simulink model "LQG"  (R2023a)
settings: Solver=FixedStepDiscrete  StartTime=0.0  StopTime=input_settings.flight_time  FixedStep=input_settings.dt  RelTol=1e-3
undefined symbols (not defined in the file): control_surface_mapping, DiscIntNeverNeededParam, Discrete, input_settings, linear_sys, LQR_gain, Rn, saturation_deflection_rate, sys_kf, Time
libraries: ctrlSharedLib x1
settings Model: Creator=sjd320  LastModifiedBy=sduess
settings DebuggingCC: UnconnectedInputMsg=warning  UnconnectedOutputMsg=warning  UnconnectedLineMsg=warning
settings ModelReferenceCC: EnableRefExpFcnMdlSchedulingChecks=on
settings RTWCC: DLArmComputeVersion=19.05

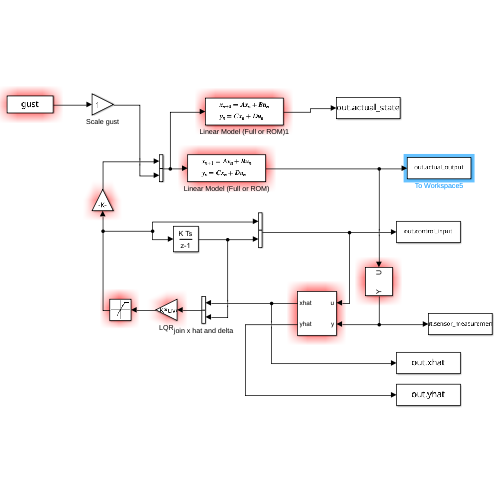
[thumbnail: Simulink's stored preview of the top-level diagram]
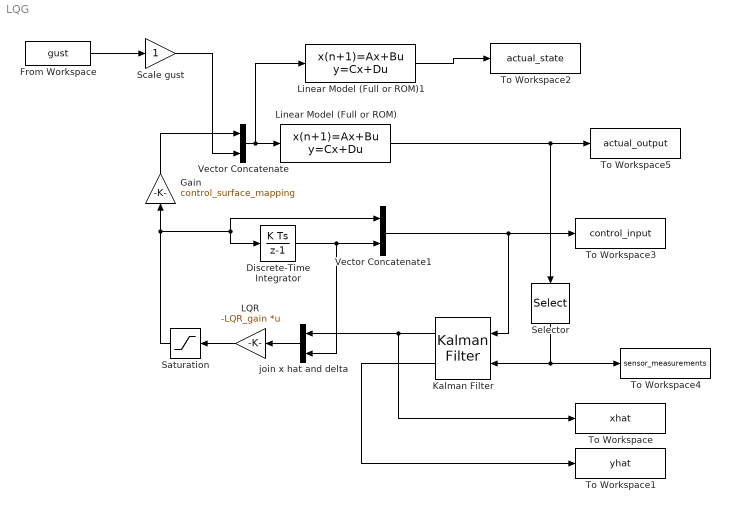
== system LQG ==
  Discrete-Time Integrator : DiscreteIntegrator  SampleTime=-1  ICPrevOutput=DiscIntNeverNeededParam  ICPrevScaledInput=DiscIntNeverNeededParam
  From Workspace : FromWorkspace  VariableName=gust  SampleTime=-1
  Gain : Gain  Gain=control_surface_mapping
  Kalman Filter : ctrlSharedLib/Kalman Filter  TimeDomain=Discrete-Time  UseCurrentEstimator=on  ModelSource=Individual A, B, C, D matrices  ModelSourceVariable=ss(0.95,1,1,0,1)  A=sys_kf.A  B=sys_kf.B(:,1:end-1)  C=sys_kf.C  D=sys_kf.D(:,1:end-1)  NumberOfStates=1  NumberOfInputs=1  NumberOfOutputs=1  InitialEstimateSource=Dialog  X0=0  P0=10  UseK=off  UseGH=on  NumberOfProcessNoiseInputs=1  G=sys_kf.B(:,end)  TimeInvariantG=on  H=sys_kf.D(:,end)  TimeInvariantH=on  Q=Qn  TimeInvariantQ=on  R=Rn  TimeInvariantR=on  N=0  TimeInvariantN=on  AddInputPort=on  AddEnablePort=off  OutputEstimatedY=on  OutputP=off  Ts=-1
  LQR : Gain  Gain=-LQR_gain  Multiplication=Matrix(K*u) (u vector)
  Linear Model (Full or ROM) : DiscreteStateSpace  A=linear_sys.A  B=linear_sys.B  C=linear_sys.C  D=linear_sys.D  SampleTime=input_settings.dt
  Linear Model (Full or ROM)1 : DiscreteStateSpace  A=linear_sys.A  B=linear_sys.B  C=eye(size(linear_sys.A,1))  D=linear_sys.B.*0.  SampleTime=input_settings.dt
  Saturation : Saturate  UpperLimit=saturation_deflection_rate  LowerLimit=-saturation_deflection_rate
  Scale gust : Gain
  Selector : Selector  InputPortWidth=size(linear_sys.C,1)  IndexOptions=Index vector (dialog)  Indices=input_settings.sensors  OutputSizes=1
  To Workspace : ToWorkspace  VariableName=xhat  SaveFormat=Timeseries  SampleTime=-1
  To Workspace1 : ToWorkspace  VariableName=yhat  SaveFormat=Timeseries  SampleTime=-1
  To Workspace2 : ToWorkspace  VariableName=actual_state  SaveFormat=Timeseries  SampleTime=-1
  To Workspace3 : ToWorkspace  VariableName=control_input  SaveFormat=Timeseries  SampleTime=-1
  To Workspace4 : ToWorkspace  VariableName=sensor_measurements  SaveFormat=Timeseries  SampleTime=-1
  To Workspace5 : ToWorkspace  VariableName=actual_output  SaveFormat=Timeseries  SampleTime=-1
  Vector Concatenate : Concatenate
  Vector Concatenate1 : Concatenate
  join x hat and delta : Concatenate
  wires:
  From Workspace/1 -> Scale gust/1
  Scale gust/1 -> Vector Concatenate/2
  Linear Model (Full or ROM)/1 -> To Workspace5/1, Selector/1
  LQR/1 -> Saturation/1
  Saturation/1 -> Vector Concatenate1/1, Discrete-Time Integrator/1, Gain/1
  Gain/1 -> Vector Concatenate/1
  Vector Concatenate1/1 -> To Workspace3/1, Kalman Filter/1
  Discrete-Time Integrator/1 -> join x hat and delta/2, Vector Concatenate1/2
  join x hat and delta/1 -> LQR/1
  Kalman Filter/1 -> To Workspace/1, join x hat and delta/1
  Kalman Filter/2 -> To Workspace1/1
  Selector/1 -> To Workspace4/1, Kalman Filter/2
  Vector Concatenate/1 -> Linear Model (Full or ROM)1/1, Linear Model (Full or ROM)/1
  Linear Model (Full or ROM)1/1 -> To Workspace2/1
